simulink model "battery_manager"  (R2020b)
settings: Solver=FixedStepDiscrete  StartTime=0.0  StopTime=10.0  FixedStep=ContIntTime  RelTol=1e-3
undefined symbols (not defined in the file): packCapacity_kWh, packVoltage_V, PowerThreshold, SmoothnessOfTheStop, TimeToStop, VoltageThreshold
libraries: simulink x2
settings Model: DataDictionary=battery_manager.sldd  Creator=Dmitry  LastModifiedBy=Dmitry
settings DebuggingCC: UnderSpecifiedDimensionMsg=warning

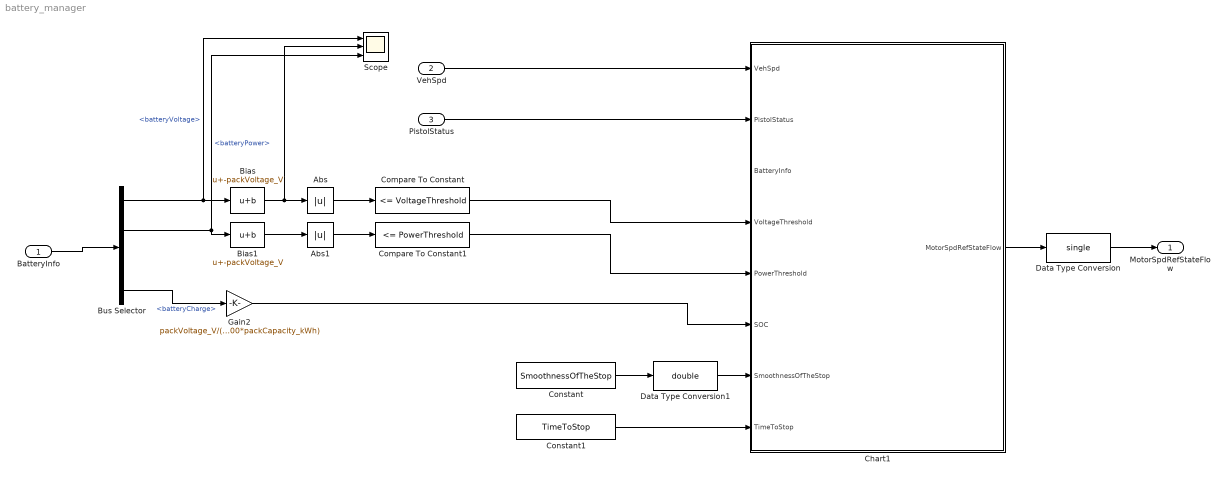
== system battery_manager ==
  BatteryInfo : Inport  OutDataTypeStr=Bus: BatteryInfo
  VehSpd : Inport  Port=2  OutDataTypeStr=single
  PistolStatus : Inport  Port=3  OutDataTypeStr=Enum: EnumPistSt
  Abs : Abs
  Abs1 : Abs
  Bias : Bias  Bias=-packVoltage_V
  Bias1 : Bias  Bias=-packVoltage_V
  Bus Selector : BusSelector  OutputSignals=batteryVoltage,batteryPower,batteryCurrent,batteryCharge
  Chart1 : Stateflow chart  TreatAsAtomicUnit=on
  Compare To Constant : simulink/Logic and Bit Operations/Compare To Constant  relop=<=  const=VoltageThreshold  OutDataTypeStr=boolean
  Compare To Constant1 : simulink/Logic and Bit Operations/Compare To Constant  relop=<=  const=PowerThreshold  OutDataTypeStr=boolean
  Constant : Constant  Value=SmoothnessOfTheStop
  Constant1 : Constant  Value=TimeToStop
  Data Type Conversion : DataTypeConversion  OutDataTypeStr=single
  Data Type Conversion1 : DataTypeConversion  OutDataTypeStr=double
  Gain2 : Gain  Gain=packVoltage_V/(1000*packCapacity_kWh)
  Scope : Scope  NumInputPorts=3
  MotorSpdRefStateFlow : Outport  OutDataTypeStr=single
  wires:
  Chart1/1(MotorSpdRefStateFlow) -> Data Type Conversion/1
  VehSpd/1 -> Chart1/1(VehSpd)
  PistolStatus/1 -> Chart1/2(PistolStatus)
  BatteryInfo/1 -> Bus Selector/1
  Bus Selector/1 -> Scope/1, Bias/1  "<batteryVoltage>"
  Bias/1 -> Scope/2, Abs/1
  Abs/1 -> Compare To Constant/1
  Bus Selector/2 -> Scope/3, Bias1/1  "<batteryPower>"
  Bias1/1 -> Abs1/1
  Abs1/1 -> Compare To Constant1/1
  Bus Selector/4 -> Gain2/1  "<batteryCharge>"
  Gain2/1 -> Chart1/6(SOC)
  Compare To Constant/1 -> Chart1/4(VoltageThreshold)
  Compare To Constant1/1 -> Chart1/5(PowerThreshold)
  Constant/1 -> Data Type Conversion1/1
  Constant1/1 -> Chart1/8(TimeToStop)
  Data Type Conversion/1 -> MotorSpdRefStateFlow/1
  Data Type Conversion1/1 -> Chart1/7(SmoothnessOfTheStop)

== stateflow chart battery_manager/Chart1 ==
  state DriveSmooth
    entry:
    OnFault=0;
    count=0
    state a
      entry:
      MotorSpdRefStateFlow=MotorSpdRefStateFlow+k;
    state b1
      entry:
    (default) -> DriveSmooth.a
    b1 -> DriveSmooth.a : after(TimeToStop/SmoothnessOfTheStop,sec)
    DriveSmooth.a -> b1 : {count=count+1}
  state Off
    entry:
    k=1/SmoothnessOfTheStop;
    (default) -> (junction 100) : % Initialization
    (junction 100) -> (junction 101) [order 1] : [VoltageThreshold==1||PowerThreshold==0||SOC<0.05]
    (junction 100) -> (junction 102) [order 2] : {fault=0;}
    (junction 101) -> (junction 103) : {fault=1;}
    (junction 103) -> (junction 102)
    (junction 102) -> (junction 104)
  state On
  state Charge
    entry:
    fault=0;
    during:
  state Drive
    entry:
    during:
  state Fault
    entry:
    OnFault=1;
    count=0;
    state a
      entry:
      MotorSpdRefStateFlow=MotorSpdRefStateFlow-k;
    state b
      entry:
    (default) -> Fault.a
    Fault.a -> b : {count=count+1}
    b -> Fault.a : after(TimeToStop/SmoothnessOfTheStop,sec)
  On -> DriveSmooth [order 3] : [OnFault==1]
  DriveSmooth -> On : [count==SmoothnessOfTheStop]{count=0}
  (default) -> Off
  Off -> On [order 2] : [fault==0]
  On -> Charge [order 2] : [PistolStatus==EnumPistSt.PluggedIn]
  Charge -> On : [PistolStatus==EnumPistSt.UnPlugged&&SOC>0.2]
  Drive -> On [order 1] : [VehSpd == 0]
  On -> Drive [order 1] : [fault==0&&VehSpd>0]
  Fault -> Charge [order 1] : [PistolStatus==EnumPistSt.PluggedIn]
  Off -> Fault [order 1] : after(0.01,sec)[fault==1&&OnFault==0]
  Fault -> Off [order 2] : [count==SmoothnessOfTheStop]{MotorSpdRefStateFlow=0}
  Drive -> Fault [order 2] : [SOC<0.1]
  data: MotorSpdRefStateFlow output double =1; fault local double =2; k local double; VehSpd input; PistolStatus input; BatteryInfo input; VoltageThreshold input; PowerThreshold input; SOC input =100; OnFault local =0; SmoothnessOfTheStop input; TimeToStop input; count local =0
